simulink model "TemplateLgV2"  (Simulink 7.3)
settings: Solver=ode5  StartTime=0.0  StopTime=inf  FixedStep=0.1  RelTol=1e-3
undefined symbols (not defined in the file): eta1_0_real, v1_0_real, velocitySatValues1
libraries: simulink x23, dspmtrx3 x18, marine_gnc x9, dspindex x5, simulink_extras x1, dspinverses x1
(part 4 of 4)

== system TemplateLgV2/Main Subsystems/Guidance/Line-Of-Sight Path-Following/Line-Of-Sight/LOS heading/psi_los^qs = psi_los^sq ==
  epsilon_n : Inport
  Delta : Inport  Port=2
  epsilon_n^s : Inport  Port=3
  epsilon_n^q : Inport  Port=4
  epsilon_n^qs : Inport  Port=5
  ( )^2 : Math  Operator=square  OutDataType=fixdt(1, 16)  OutScaling=2^0  SaturateOnIntegerOverflow=on
  2 : Gain  Gain=2  ParameterDataType=fixdt(1, 16)  ParameterScaling=2^0  OutDataType=fixdt(1, 16)  OutScaling=2^0
  Add : Sum  Inputs=|++  OutDataType=fixdt(1, 16)  OutScaling=2^-10
  Delta^2 : Math  Operator=square  OutDataType=fixdt(1, 16)  OutScaling=2^0  SaturateOnIntegerOverflow=on
  Divide : Product  Inputs=*/  OutDataType=fixdt(1, 16)  OutScaling=2^-10
  Divide1 : Product  Inputs=*/  OutDataType=fixdt(1, 16)  OutScaling=2^-10
  Product : Product  Inputs=4  Multiplication=Matrix(*)  OutDataType=fixdt(1, 16)  OutScaling=2^0  RndMeth=Zero
  Product1 : Product  Multiplication=Matrix(*)  OutDataType=fixdt(1, 16)  OutScaling=2^0  RndMeth=Zero
  Subtract : Sum  Inputs=|+-  OutDataType=fixdt(1, 16)  OutScaling=2^-10
  epsilon_n^2 : Math  Operator=square  OutDataType=fixdt(1, 16)  OutScaling=2^0  SaturateOnIntegerOverflow=on
  psi_los^qs : Outport
  wires:
  2/1 -> Divide/1
  Divide1/1 -> Subtract/2
  Product1/1 -> Divide1/1
  epsilon_n^qs/1 -> Product1/2
  ( )^2/1 -> Divide/2
  Delta^2/1 -> Add/1
  Add/1 -> Divide1/2, ( )^2/1
  epsilon_n^2/1 -> Add/2
  Product/1 -> 2/1
  epsilon_n^q/1 -> Product/4
  epsilon_n^s/1 -> Product/3
  epsilon_n/1 -> epsilon_n^2/1, Product/2
  Delta/1 -> Product1/1, Delta^2/1, Product/1
  Divide/1 -> Subtract/1
  Subtract/1 -> psi_los^qs/1

== system TemplateLgV2/Main Subsystems/Guidance/Line-Of-Sight Path-Following/Line-Of-Sight/LOS heading/psi_los^s eq ==
  epsilon_n : Inport
  Delta : Inport  Port=2
  psi_d^s : Inport  Port=3
  epsilon_n^s : Inport  Port=4
  Add : Sum  Inputs=|++  OutDataType=fixdt(1, 16)  OutScaling=2^-10
  Delta^2 : Math  Operator=square  OutDataType=fixdt(1, 16)  OutScaling=2^0  SaturateOnIntegerOverflow=on
  Divide : Product  Inputs=*/  OutDataType=fixdt(1, 16)  OutScaling=2^-10
  Product : Product  OutDataType=fixdt(1, 16)  OutScaling=2^0  RndMeth=Zero
  Subtract : Sum  Inputs=|+-  OutDataType=fixdt(1, 16)  OutScaling=2^-10
  epsilon_n^2 : Math  Operator=square  OutDataType=fixdt(1, 16)  OutScaling=2^0  SaturateOnIntegerOverflow=on
  psi_los^s : Outport
  wires:
  Delta/1 -> Divide/1, Delta^2/1
  Delta^2/1 -> Add/1
  Add/1 -> Divide/2
  epsilon_n^2/1 -> Add/2
  epsilon_n/1 -> epsilon_n^2/1
  Subtract/1 -> psi_los^s/1
  Product/1 -> Subtract/2
  psi_d^s/1 -> Subtract/1
  epsilon_n^s/1 -> Product/2
  Divide/1 -> Product/1

== system TemplateLgV2/Main Subsystems/Guidance/Line-Of-Sight Path-Following/Line-Of-Sight/LOS heading/psi_los^s^2 eq ==
  epsilon_n : Inport
  Delta : Inport  Port=2
  epsilon_n^s : Inport  Port=3
  psi_d¨^s^2 : Inport  Port=4
  epsilon_n^s^2 : Inport  Port=5
  ( )^2 : Math  Operator=square  OutDataType=fixdt(1, 16)  OutScaling=2^0  SaturateOnIntegerOverflow=on
  (epsilon_n^s)^2 : Math  Operator=square  OutDataType=fixdt(1, 16)  OutScaling=2^0  SaturateOnIntegerOverflow=on
  2 : Gain  Gain=2  ParameterDataType=fixdt(1, 16)  ParameterScaling=2^0  OutDataType=fixdt(1, 16)  OutScaling=2^0
  Add : Sum  Inputs=|++  OutDataType=fixdt(1, 16)  OutScaling=2^-10
  Delta^2 : Math  Operator=square  OutDataType=fixdt(1, 16)  OutScaling=2^0  SaturateOnIntegerOverflow=on
  Divide : Product  Inputs=*/  OutDataType=fixdt(1, 16)  OutScaling=2^-10
  Divide1 : Product  Inputs=*/  OutDataType=fixdt(1, 16)  OutScaling=2^-10
  Product : Product  Inputs=3  Multiplication=Matrix(*)  OutDataType=fixdt(1, 16)  OutScaling=2^0  RndMeth=Zero
  Product1 : Product  Multiplication=Matrix(*)  OutDataType=fixdt(1, 16)  OutScaling=2^0  RndMeth=Zero
  Sum : Sum  Inputs=++-  OutDataType=fixdt(1, 16)  OutScaling=2^-10
  epsilon_n^2 : Math  Operator=square  OutDataType=fixdt(1, 16)  OutScaling=2^0  SaturateOnIntegerOverflow=on
  psi_los^s^2 : Outport
  wires:
  epsilon_n^s^2/1 -> Product1/2
  epsilon_n^s/1 -> (epsilon_n^s)^2/1
  2/1 -> Divide/1
  Divide1/1 -> Sum/3
  Product1/1 -> Divide1/1
  ( )^2/1 -> Divide/2
  Delta^2/1 -> Add/1
  Add/1 -> Divide1/2, ( )^2/1
  epsilon_n^2/1 -> Add/2
  Product/1 -> 2/1
  (epsilon_n^s)^2/1 -> Product/3
  epsilon_n/1 -> epsilon_n^2/1, Product/2
  Delta/1 -> Product1/1, Delta^2/1, Product/1
  Divide/1 -> Sum/2
  psi_d¨^s^2/1 -> Sum/1
  Sum/1 -> psi_los^s^2/1

== system TemplateLgV2/Main Subsystems/Guidance/Line-Of-Sight Path-Following/Line-Of-Sight/Position error signals/R_2 ==
  psi_d : Inport
  Mux : Mux
  R11 : Trigonometry  Operator=cos
  R12 : Gain  Gain=-1  ParameterDataType=fixdt(1, 16)  ParameterScaling=2^0  OutDataType=fixdt(1, 16)  OutScaling=2^0
  R21 : Trigonometry
  R22 : Gain  ParameterDataType=fixdt(1, 16)  ParameterScaling=2^0  OutDataType=fixdt(1, 16)  OutScaling=2^0
  R_2(psi_d) : Reshape  OutputDimensionality=Customize  OutputDimensions=[2,2]
  R_2 : Outport
  wires:
  R22/1 -> Mux/4
  R12/1 -> Mux/3
  R11/1 -> R22/1, Mux/1
  psi_d/1 -> R11/1, R21/1
  R21/1 -> Mux/2, R12/1
  Mux/1 -> R_2(psi_d)/1
  R_2(psi_d)/1 -> R_2/1

== system TemplateLgV2/Main Subsystems/Guidance/Line-Of-Sight Path-Following/Line-Of-Sight/Position error signals/S_2 ==
  psi_d^s : Inport
  0 : Constant  Value=0  OutDataType=fixdt(1, 16)  OutScaling=2^0
  Mux : Mux
  S12 : Gain  Gain=-1  ParameterDataType=fixdt(1, 16)  ParameterScaling=2^0  OutDataType=fixdt(1, 16)  OutScaling=2^0
  S_2(psi_d^s) : Reshape  OutputDimensionality=Customize  OutputDimensions=[2,2]
  S_2 : Outport
  wires:
  0/1 -> Mux/1, Mux/4
  S12/1 -> Mux/3
  psi_d^s/1 -> Mux/2, S12/1
  Mux/1 -> S_2(psi_d^s)/1
  S_2(psi_d^s)/1 -> S_2/1

== system TemplateLgV2/Main Subsystems/Guidance/Line-Of-Sight Path-Following/Line-Of-Sight/Position error signals/S_2(psi_d^s^2) ==
  psi_d^s^2 : Inport
  0 : Constant  Value=0  OutDataType=fixdt(1, 16)  OutScaling=2^0
  Mux : Mux
  S12 : Gain  Gain=-1  ParameterDataType=fixdt(1, 16)  ParameterScaling=2^0  OutDataType=fixdt(1, 16)  OutScaling=2^0
  S_2(psi_d^s^2) : Reshape  OutputDimensionality=Customize  OutputDimensions=[2,2]
  S_2 : Outport
  wires:
  S_2(psi_d^s^2)/1 -> S_2/1
  Mux/1 -> S_2(psi_d^s^2)/1
  psi_d^s^2/1 -> S12/1, Mux/2
  S12/1 -> Mux/3
  0/1 -> Mux/4, Mux/1

== system TemplateLgV2/Main Subsystems/Guidance/Line-Of-Sight Path-Following/Line-Of-Sight/Position error signals/epsilon^qs = epsilon^sq ==
  R_2^T : Inport
  S_2^T : Inport  Port=2
  Product1 : Product  Multiplication=Matrix(*)  OutDataType=fixdt(1, 16)  OutScaling=2^0  RndMeth=Zero
  epsilon^qs : Outport
  wires:
  R_2^T/1 -> Product1/2
  S_2^T/1 -> Product1/1
  Product1/1 -> epsilon^qs/1

== system TemplateLgV2/Main Subsystems/Guidance/Line-Of-Sight Path-Following/Line-Of-Sight/Position error signals/epsilon^s eq ==
  q - p_d : Inport
  R_2^T : Inport  Port=2
  S_2^T : Inport  Port=3
  p_d^s : Inport  Port=4
  Product : Product  Inputs=3  Multiplication=Matrix(*)  OutDataType=fixdt(1, 16)  OutScaling=2^0  RndMeth=Zero
  Product1 : Product  Multiplication=Matrix(*)  OutDataType=fixdt(1, 16)  OutScaling=2^0  RndMeth=Zero
  Subtract1 : Sum  Inputs=+-  OutDataType=fixdt(1, 16)  OutScaling=2^-10
  epsilon^s : Outport
  wires:
  q - p_d/1 -> Product/3
  Subtract1/1 -> epsilon^s/1
  Product1/1 -> Subtract1/2
  Product/1 -> Subtract1/1
  p_d^s/1 -> Product1/2
  R_2^T/1 -> Product1/1, Product/2
  S_2^T/1 -> Product/1

== system TemplateLgV2/Main Subsystems/Guidance/Line-Of-Sight Path-Following/Line-Of-Sight/Position error signals/epsilon^s^2 eq ==
  q - p_d : Inport
  p_d^s : Inport  Port=2
  R_2^T : Inport  Port=3
  S_2^T : Inport  Port=4
  S_2(psi_d^s^2)^T : Inport  Port=5
  p_d^s^2 : Inport  Port=6
  2 : Gain  Gain=2  ParameterDataType=fixdt(1, 16)  ParameterScaling=2^0  OutDataType=fixdt(1, 16)  OutScaling=2^0
  Add : Sum  OutDataType=fixdt(1, 16)  OutScaling=2^-10
  Gain : Gain  ParameterDataType=fixdt(1, 16)  ParameterScaling=2^0  OutDataType=fixdt(1, 16)  OutScaling=2^0
  Product : Product  Multiplication=Matrix(*)  OutDataType=fixdt(1, 16)  OutScaling=2^0  RndMeth=Zero
  Product1 : Product  Inputs=3  Multiplication=Matrix(*)  OutDataType=fixdt(1, 16)  OutScaling=2^0  RndMeth=Zero
  Product2 : Product  Inputs=3  Multiplication=Matrix(*)  OutDataType=fixdt(1, 16)  OutScaling=2^0  RndMeth=Zero
  Product3 : Product  Multiplication=Matrix(*)  OutDataType=fixdt(1, 16)  OutScaling=2^0  RndMeth=Zero
  Sum : Sum  Inputs=+--  OutDataType=fixdt(1, 16)  OutScaling=2^-10
  epsilon^s^2 : Outport
  wires:
  Product3/1 -> Sum/3
  p_d^s^2/1 -> Product3/2
  p_d^s/1 -> Product2/3
  2/1 -> Sum/2
  Product1/1 -> Sum/1
  q - p_d/1 -> Product1/3
  R_2^T/1 -> Product3/1, Product2/2, Product1/2
  Add/1 -> Product1/1
  Product/1 -> Add/2
  S_2^T/1 -> Product/2, Product2/1, Product/1
  S_2(psi_d^s^2)^T/1 -> Add/1
  Gain/1 -> epsilon^s^2/1
  Product2/1 -> 2/1
  Sum/1 -> Gain/1

== system TemplateLgV2/Main Subsystems/Guidance/Line-Of-Sight Path-Following/Path/Ellipse path/p_d eq ==
  s : Inport
  r_x : Inport  Port=2
  r_y : Inport  Port=3
  origo_x : Inport  Port=4
  origo_y : Inport  Port=5
  k : Inport  Port=6
  Add : Sum  OutDataType=fixdt(1, 16)  OutScaling=2^-10
  Add1 : Sum  OutDataType=fixdt(1, 16)  OutScaling=2^-10
  Mux1 : Mux  Inputs=2
  Product : Product  OutDataType=fixdt(1, 16)  OutScaling=2^0  RndMeth=Zero
  Product1 : Product  OutDataType=fixdt(1, 16)  OutScaling=2^0  RndMeth=Zero
  Product2 : Product  OutDataType=fixdt(1, 16)  OutScaling=2^0  RndMeth=Zero
  cos(s) : Trigonometry  Operator=cos
  sin(s) : Trigonometry
  p_d : Outport
  wires:
  Product2/1 -> sin(s)/1, cos(s)/1
  k/1 -> Product2/2
  s/1 -> Product2/1
  Add1/1 -> Mux1/2
  Product1/1 -> Add1/1
  Product/1 -> Add/1
  origo_y/1 -> Add1/2
  origo_x/1 -> Add/2
  Mux1/1 -> p_d/1
  r_y/1 -> Product1/1
  r_x/1 -> Product/1
  Add/1 -> Mux1/1
  sin(s)/1 -> Product1/2
  cos(s)/1 -> Product/2

== system TemplateLgV2/Main Subsystems/Guidance/Line-Of-Sight Path-Following/Path/Ellipse path/p_d^s eq ==
  s : Inport
  r_x : Inport  Port=2
  r_y : Inport  Port=3
  k : Inport  Port=4
  Gain : Gain  Gain=-1  ParameterDataType=fixdt(1, 16)  ParameterScaling=2^0  OutDataType=fixdt(1, 16)  OutScaling=2^0
  Mux1 : Mux  Inputs=2
  Product : Product  Inputs=3  OutDataType=fixdt(1, 16)  OutScaling=2^0  RndMeth=Zero
  Product1 : Product  Inputs=3  OutDataType=fixdt(1, 16)  OutScaling=2^0  RndMeth=Zero
  Product2 : Product  OutDataType=fixdt(1, 16)  OutScaling=2^0  RndMeth=Zero
  cos(s) : Trigonometry  Operator=cos
  sin(s) : Trigonometry
  p_d^s : Outport
  wires:
  Product2/1 -> sin(s)/1, cos(s)/1
  k/1 -> Product/3, Product1/3, Product2/2
  Mux1/1 -> p_d^s/1
  r_y/1 -> Product1/1
  r_x/1 -> Product/1
  Product1/1 -> Mux1/2
  Gain/1 -> Mux1/1
  Product/1 -> Gain/1
  cos(s)/1 -> Product1/2
  sin(s)/1 -> Product/2
  s/1 -> Product2/1

== system TemplateLgV2/Main Subsystems/Guidance/Line-Of-Sight Path-Following/Path/Ellipse path/p_d^s^2 eq ==
  s : Inport
  r_x : Inport  Port=2
  r_y : Inport  Port=3
  k : Inport  Port=4
  Gain : Gain  Gain=-1  ParameterDataType=fixdt(1, 16)  ParameterScaling=2^0  OutDataType=fixdt(1, 16)  OutScaling=2^0
  Gain1 : Gain  Gain=-1  ParameterDataType=fixdt(1, 16)  ParameterScaling=2^0  OutDataType=fixdt(1, 16)  OutScaling=2^0
  Math Function : Math  Operator=square  OutDataType=fixdt(1, 16)  OutScaling=2^0  SaturateOnIntegerOverflow=on
  Mux2 : Mux  Inputs=2
  Product : Product  Inputs=3  OutDataType=fixdt(1, 16)  OutScaling=2^0  RndMeth=Zero
  Product1 : Product  Inputs=3  OutDataType=fixdt(1, 16)  OutScaling=2^0  RndMeth=Zero
  Product2 : Product  OutDataType=fixdt(1, 16)  OutScaling=2^0  RndMeth=Zero
  cos(s) : Trigonometry  Operator=cos
  sin(s) : Trigonometry
  p_d^s^2 : Outport
  wires:
  Math Function/1 -> Product/3, Product1/3
  Product2/1 -> sin(s)/1, cos(s)/1
  s/1 -> Product2/1
  k/1 -> Math Function/1, Product2/2
  r_x/1 -> Product/1
  r_y/1 -> Product1/1
  Mux2/1 -> p_d^s^2/1
  sin(s)/1 -> Product1/2
  cos(s)/1 -> Product/2
  Gain1/1 -> Mux2/2
  Product1/1 -> Gain1/1
  Gain/1 -> Mux2/1
  Product/1 -> Gain/1

== system TemplateLgV2/Main Subsystems/Guidance/Line-Of-Sight Path-Following/Path/Ellipse path/p_d^s^3 eq ==
  s : Inport
  r_x : Inport  Port=2
  r_y : Inport  Port=3
  k : Inport  Port=4
  Constant : Constant  Value=3  OutDataType=fixdt(1, 16)  OutScaling=2^0
  Gain : Gain  Gain=-1  ParameterDataType=fixdt(1, 16)  ParameterScaling=2^0  OutDataType=fixdt(1, 16)  OutScaling=2^0
  Math Function : Math  Operator=pow  OutDataType=fixdt(1, 16)  OutScaling=2^0  SaturateOnIntegerOverflow=on
  Mux3 : Mux  Inputs=2
  Product : Product  Inputs=3  OutDataType=fixdt(1, 16)  OutScaling=2^0  RndMeth=Zero
  Product1 : Product  Inputs=3  OutDataType=fixdt(1, 16)  OutScaling=2^0  RndMeth=Zero
  Product2 : Product  OutDataType=fixdt(1, 16)  OutScaling=2^0  RndMeth=Zero
  cos(s)3 : Trigonometry  Operator=cos
  sin(s)3 : Trigonometry
  p_d^s^3 : Outport
  wires:
  Math Function/1 -> Product/3, Product1/3
  Constant/1 -> Math Function/2
  Product2/1 -> cos(s)3/1, sin(s)3/1
  s/1 -> Product2/1
  k/1 -> Math Function/1, Product2/2
  r_y/1 -> Product1/1
  r_x/1 -> Product/1
  sin(s)3/1 -> Product/2
  cos(s)3/1 -> Product1/2
  Product/1 -> Mux3/1
  Mux3/1 -> p_d^s^3/1
  Gain/1 -> Mux3/2
  Product1/1 -> Gain/1

== system TemplateLgV2/Main Subsystems/Guidance/Line-Of-Sight Path-Following/Path/Ellipse path/|p_d^s| eq ==
  p_d^s : Inport
  Product : Product  Multiplication=Matrix(*)  OutDataType=fixdt(1, 16)  OutScaling=2^0  RndMeth=Zero
  p_d^s^T : dspmtrx3/Transpose  SystemSampleTime=-1  Hermitian=off  overflowFlag=off
  sqrt : Math  Operator=sqrt  OutDataType=fixdt(1, 16)  OutScaling=2^0  SaturateOnIntegerOverflow=on
  |p_d^s| : Outport
  wires:
  p_d^s^T/1 -> Product/1
  Product/1 -> sqrt/1
  sqrt/1 -> |p_d^s|/1
  p_d^s/1 -> p_d^s^T/1, Product/2

== system TemplateLgV2/Main Subsystems/Guidance/Line-Of-Sight Path-Following/Path/Path Switch workaround + limiter/Limiter ==
  p_d : Inport  OutDataType=sfix(16)  OutScaling=2^0
  Demux : Demux  Outputs=2
  Mux1 : Mux  Inputs=2
  Saturation x : simulink/Discontinuities/Saturation Dynamic  SystemSampleTime=-1  OutMin=[]  OutMax=[]  OutDataTypeStr=Inherit: Same as second input  OutDataType=fixdt(1, 16)  OutScaling=2^-10  DoSatur=off
  Saturation y : simulink/Discontinuities/Saturation Dynamic  SystemSampleTime=-1  OutMin=[]  OutMax=[]  OutDataTypeStr=Inherit: Same as second input  OutDataType=fixdt(1, 16)  OutScaling=2^-10  DoSatur=off
  sat_p_d : Outport  PortDimensions=2  OutDataType=sfix(16)  OutScaling=2^0
  wires:
  Saturation y/1 -> Mux1/2
  Saturation x/1 -> Mux1/1
  Demux/2 -> Saturation y/2
  Demux/1 -> Saturation x/2
  p_d/1 -> Demux/1
  Mux1/1 -> sat_p_d/1
  [xdmax] -> Saturation x/1
  [xdmin] -> Saturation x/3
  [ydmax] -> Saturation y/1
  [ydmin] -> Saturation y/3

== system TemplateLgV2/Main Subsystems/Guidance/Line-Of-Sight Path-Following/Path/Path Switch workaround + limiter/p_d selcetor ==
  note: Path Selector == 1: Linear path
      | Path Selector == 0: Ellipse path
  Path Selector : Inport  OutDataType=fixdt(1, 16)  OutScaling=2^0
  Add : Sum  OutDataType=fixdt(1, 16)  OutScaling=2^-10
  Constant : Constant  OutDataType=fixdt(1, 16)  OutScaling=2^0
  Product : Product  OutDataType=fixdt(1, 16)  OutScaling=2^0  RndMeth=Zero
  Product1 : Product  OutDataType=fixdt(1, 16)  OutScaling=2^0  RndMeth=Zero
  Subract : Sum  Inputs=+-  OutDataType=fixdt(1, 16)  OutScaling=2^-10
  p_d : Outport
  wires:
  Add/1 -> p_d/1
  Path Selector/1 -> Product/2, Subract/2  "chosen path"
  Constant/1 -> Subract/1
  Product/1 -> Add/1
  Subract/1 -> Product1/2
  Product1/1 -> Add/2
  [pdLinear] -> Product/1
  [pdEllipse] -> Product1/1

== system TemplateLgV2/Main Subsystems/Guidance/Line-Of-Sight Path-Following/Path/Path Switch workaround + limiter/p_d^s selcetor ==
  note: Path Selector == 1: Linear path
      | Path Selector == 0: Ellipse path
  Path Selector : Inport  OutDataType=fixdt(1, 16)  OutScaling=2^0
  Add : Sum  OutDataType=fixdt(1, 16)  OutScaling=2^-10
  Constant : Constant  OutDataType=fixdt(1, 16)  OutScaling=2^0
  Product : Product  OutDataType=fixdt(1, 16)  OutScaling=2^0  RndMeth=Zero
  Product1 : Product  OutDataType=fixdt(1, 16)  OutScaling=2^0  RndMeth=Zero
  Subract : Sum  Inputs=+-  OutDataType=fixdt(1, 16)  OutScaling=2^-10
  p_d^s : Outport
  wires:
  [pd_sEllipse] -> Product1/1
  [pd_sLinear] -> Product/1
  Product1/1 -> Add/2
  Subract/1 -> Product1/2
  Product/1 -> Add/1
  Constant/1 -> Subract/1
  Path Selector/1 -> Subract/2, Product/2  "chosen path"
  Add/1 -> p_d^s/1

== system TemplateLgV2/Main Subsystems/Guidance/Line-Of-Sight Path-Following/Path/Path Switch workaround + limiter/p_d^s^2 selcetor ==
  note: Path Selector == 1: Linear path
      | Path Selector == 0: Ellipse path
  Path Selector : Inport  OutDataType=fixdt(1, 16)  OutScaling=2^0
  Add : Sum  OutDataType=fixdt(1, 16)  OutScaling=2^-10
  Constant : Constant  OutDataType=fixdt(1, 16)  OutScaling=2^0
  Product : Product  OutDataType=fixdt(1, 16)  OutScaling=2^0  RndMeth=Zero
  Product1 : Product  OutDataType=fixdt(1, 16)  OutScaling=2^0  RndMeth=Zero
  Subract : Sum  Inputs=+-  OutDataType=fixdt(1, 16)  OutScaling=2^-10
  p_d^s^2 : Outport
  wires:
  Add/1 -> p_d^s^2/1
  Path Selector/1 -> Product/2, Subract/2  "chosen path"
  Constant/1 -> Subract/1
  Product/1 -> Add/1
  Subract/1 -> Product1/2
  Product1/1 -> Add/2
  [pd_s_2Linear] -> Product/1
  [pd_s_2Ellipse] -> Product1/1

== system TemplateLgV2/Main Subsystems/Guidance/Line-Of-Sight Path-Following/Path/Path Switch workaround + limiter/p_d^s^3 selcetor ==
  note: Path Selector == 1: Linear path
      | Path Selector == 0: Ellipse path
  Path Selector : Inport  OutDataType=fixdt(1, 16)  OutScaling=2^0
  Add : Sum  OutDataType=fixdt(1, 16)  OutScaling=2^-10
  Constant : Constant  OutDataType=fixdt(1, 16)  OutScaling=2^0
  Product : Product  OutDataType=fixdt(1, 16)  OutScaling=2^0  RndMeth=Zero
  Product1 : Product  OutDataType=fixdt(1, 16)  OutScaling=2^0  RndMeth=Zero
  Subract : Sum  Inputs=+-  OutDataType=fixdt(1, 16)  OutScaling=2^-10
  p_d^s^3 : Outport
  wires:
  [pd_s_3Ellipse] -> Product1/1
  [pd_s_3Linear] -> Product/1
  Product1/1 -> Add/2
  Subract/1 -> Product1/2
  Product/1 -> Add/1
  Constant/1 -> Subract/1
  Path Selector/1 -> Subract/2, Product/2  "chosen path"
  Add/1 -> p_d^s^3/1

== system TemplateLgV2/Main Subsystems/Guidance/Line-Of-Sight Path-Following/Path/Path Switch workaround + limiter/p_d^s^3 selcetor1 ==
  note: Path Selector == 1: Linear path
      | Path Selector == 0: Ellipse path
  Path Selector : Inport  OutDataType=fixdt(1, 16)  OutScaling=2^0
  Add : Sum  OutDataType=fixdt(1, 16)  OutScaling=2^-10
  Constant : Constant  OutDataType=fixdt(1, 16)  OutScaling=2^0
  Product : Product  OutDataType=fixdt(1, 16)  OutScaling=2^0  RndMeth=Zero
  Product1 : Product  OutDataType=fixdt(1, 16)  OutScaling=2^0  RndMeth=Zero
  Subract : Sum  Inputs=+-  OutDataType=fixdt(1, 16)  OutScaling=2^-10
  |p_d^s| : Outport
  wires:
  Add/1 -> |p_d^s|/1
  Path Selector/1 -> Product/2, Subract/2  "chosen path"
  Constant/1 -> Subract/1
  Product/1 -> Add/1
  Subract/1 -> Product1/2
  Product1/1 -> Add/2
  [pd_sabsLinear] -> Product/1
  [pd_sabsEllipse] -> Product1/1

== system TemplateLgV2/Main Subsystems/Guidance/Line-Of-Sight Path-Following/Path/Straight path/p_d eq ==
  s : Inport
  x_1 : Inport  Port=2
  y_1 : Inport  Port=3
  x_2 : Inport  Port=4
  y_2 : Inport  Port=5
  (x_2 - x_1) * s : Product  OutDataType=fixdt(1, 16)  OutScaling=2^0  RndMeth=Zero
  (x_2 - x_1) * s + x_1 : Sum  OutDataType=fixdt(1, 16)  OutScaling=2^-10
  (y_2 - y_1) * s : Product  OutDataType=fixdt(1, 16)  OutScaling=2^0  RndMeth=Zero
  (y_2 - y_1) * s + y_1 : Sum  OutDataType=fixdt(1, 16)  OutScaling=2^-10
  Mux1 : Mux  Inputs=2
  x_2 - x_1 : Sum  Inputs=+-  OutDataType=fixdt(1, 16)  OutScaling=2^-10
  y_2 - y_1 : Sum  Inputs=+-  OutDataType=fixdt(1, 16)  OutScaling=2^-10
  p_d : Outport
  wires:
  Mux1/1 -> p_d/1
  y_1/1 -> (y_2 - y_1) * s + y_1/2, y_2 - y_1/2
  y_2/1 -> y_2 - y_1/1
  x_1/1 -> (x_2 - x_1) * s + x_1/2, x_2 - x_1/2
  x_2/1 -> x_2 - x_1/1
  s/1 -> (y_2 - y_1) * s/2, (x_2 - x_1) * s/2
  y_2 - y_1/1 -> (y_2 - y_1) * s/1
  x_2 - x_1/1 -> (x_2 - x_1) * s/1
  (y_2 - y_1) * s/1 -> (y_2 - y_1) * s + y_1/1
  (x_2 - x_1) * s/1 -> (x_2 - x_1) * s + x_1/1
  (y_2 - y_1) * s + y_1/1 -> Mux1/2
  (x_2 - x_1) * s + x_1/1 -> Mux1/1

== system TemplateLgV2/Main Subsystems/Guidance/Line-Of-Sight Path-Following/Path/Straight path/p_d^s eq ==
  x_1 : Inport
  y_1 : Inport  Port=2
  x_2 : Inport  Port=3
  y_2 : Inport  Port=4
  Mux1 : Mux  Inputs=2
  x_2 - x_1 : Sum  Inputs=+-  OutDataType=fixdt(1, 16)  OutScaling=2^-10
  y_2 - y_1 : Sum  Inputs=+-  OutDataType=fixdt(1, 16)  OutScaling=2^-10
  p_d^s : Outport
  wires:
  y_1/1 -> y_2 - y_1/2
  y_2/1 -> y_2 - y_1/1
  x_1/1 -> x_2 - x_1/2
  x_2/1 -> x_2 - x_1/1
  y_2 - y_1/1 -> Mux1/2
  x_2 - x_1/1 -> Mux1/1
  Mux1/1 -> p_d^s/1

== system TemplateLgV2/Main Subsystems/Guidance/Line-Of-Sight Path-Following/Path/Straight path/|p_d^s| eq ==
  p_d^s : Inport
  Product : Product  Multiplication=Matrix(*)  OutDataType=fixdt(1, 16)  OutScaling=2^0  RndMeth=Zero
  p_d^s^T : dspmtrx3/Transpose  SystemSampleTime=-1  Hermitian=off  overflowFlag=off
  sqrt : Math  Operator=sqrt  OutDataType=fixdt(1, 16)  OutScaling=2^0  SaturateOnIntegerOverflow=on
  |p_d^s| : Outport
  wires:
  p_d^s/1 -> Product/2, p_d^s^T/1
  sqrt/1 -> |p_d^s|/1
  Product/1 -> sqrt/1
  p_d^s^T/1 -> Product/1

== system TemplateLgV2/Main Subsystems/Naviagation/Input from SIT/u_act to tau/u_act to f_act/u_1 to f_1 VSP speed 0.3 ==
  note: Table valid for VSP speed == 0.30
  u_1 : Inport
  u_1 to f_1 : Lookup  InputValues=[-1.0000 -0.9500 -0.9000 -0.8500 -0.8000 -0.7500 -0.7000 -0.6500 -0.6000 -0.5500 -0.5000 -0.4500 -0.4000 -0.3500 -0.3000 -0.2500 -0.2000 -0.1500 -0.1000 -0.0500 0 0.0500 0.1000 0.1500 0.2000 0.2500 0.3000 0.3500 0.4000 0.4500 0.5000 0.5500 0.6000 0.6500 0.7000 0.7500 0.8000 0.8500 0.9000]  Table=[-0.6829 -0.6369 -0.5785 -0.5165 -0.4456 -0.3725 -0.3308 -0.2827 -0.2277 -0.1517 -0.1240 -0.0769 -0.0238 0.0039 0.0377 0.0635 0.1051 0.1196 0.1412 0.1721 0.1754 0.1774 0.2104 0.2200 0.2266 0.2673 0.3025 0.3486 0.3896 0.4252 0.4782 0.5164 0.5695 0.6195 0.6723 0.7449 0.7836 0.8414 0.8987 ]  LookUpMeth=Interpolation-Use End Values  OutDataType=fixdt(1, 16)  OutScaling=2^0
  f_1 : Outport
  wires:
  u_1/1 -> u_1 to f_1/1
  u_1 to f_1/1 -> f_1/1

== system TemplateLgV2/Main Subsystems/Naviagation/Input from SIT/u_act to tau/u_act to f_act/u_2 to f_2 VSP speed 0.3 ==
  note: Switching to the lookup table giving the closes value
  note: workaround setup
  note: Tables valid for VSP speed == 0.30
  u_2 : Inport
  Gain1 : Gain  Gain=3  ParameterDataType=fixdt(1, 16)  ParameterScaling=2^0  OutDataType=fixdt(1, 16)  OutScaling=2^0
  If < 0.00391 : simulink/Logic and Bit Operations/Compare To Constant  SystemSampleTime=-1  relop=<  const=-0.5  LogicOutDataTypeMode=uint8
  If < 0.06731 : simulink/Logic and Bit Operations/Compare To Constant  SystemSampleTime=-1  relop=<  const=-0.1  LogicOutDataTypeMode=uint8
  If >= 0.00391 : simulink/Logic and Bit Operations/Compare To Constant  SystemSampleTime=-1  relop=>=  const=-0.5  LogicOutDataTypeMode=uint8
  If >= 0.06731 : simulink/Logic and Bit Operations/Compare To Constant  SystemSampleTime=-1  relop=>=  const=-0.1  LogicOutDataTypeMode=uint8
  Logical Operator : Logic  AllPortsSameDT=off  OutDataTypeMode=boolean  LogicDataType=fixdt(0, 8)  OutDataTypeStr=boolean
  Multiport Switch : MultiPortSwitch  OutDataType=fixdt(1, 16)  OutScaling=2^0
  Sum : Sum  Inputs=+++  OutDataType=fixdt(1, 16)  OutScaling=2^0
  Sum1 : Sum  Inputs=|++  OutDataType=fixdt(1, 16)  OutScaling=2^0
  u_2 < -0.1 && u_2 >= -0.2 : Lookup  InputValues=|  Table=|  LookUpMeth=Interpolation-Use End Values  OutDataType=fixdt(1, 16)  OutScaling=2^0
      InputValues=|
      | [-0.2000
      |    -0.1500
      |    -0.1000]
      Table=|
      | [-0.0105
      |     0.0226
      |     0.0673]
  u_2 < -0.5 : Lookup  InputValues=|  Table=|  LookUpMeth=Interpolation-Use End Values  OutDataType=fixdt(1, 16)  OutScaling=2^0
      InputValues=|
      | [-1.0000
      |    -0.9500
      |    -0.9000
      |    -0.8500
      |    -0.8000
      |    -0.7500
      |    -0.7000
      |    -0.6500
      |    -0.6000
      |    -0.5500
      |    -0.5000]
      Table=|
      | [-0.2704
      |    -0.2259
      |    -0.1903
      |    -0.1697
      |    -0.1518
      |    -0.1234
      |    -0.0994
      |    -0.0817
      |    -0.0612
      |    -0.0123
      |     0.0039]
  u_2 => 0 : Lookup  InputValues=|  Table=|  LookUpMeth=Interpolation-Use End Values  OutDataType=fixdt(1, 16)  OutScaling=2^0
      InputValues=|
      | [0
      |     0.0500
      |     0.1000
      |     0.1500
      |     0.2000
      |     0.2500
      |     0.3000
      |     0.3500
      |     0.4000
      |     0.4500
      |     0.5000
      |     0.5500
      |     0.6000
      |     0.6500
      |     0.7000
      |     0.7500
      |     0.8000
      |     0.8500]
      Table=|
      | [0.0872
      |     0.0930
      |     0.1182
      |     0.1412
      |     0.1892
      |     0.2146
      |     0.2678
      |     0.3096
      |     0.3551
      |     0.4013
      |     0.4566
      |     0.5051
      |     0.5477
      |     0.6060
      |     0.6703
      |     0.7437
      |     0.7604
      |     0.7634]
  f_2 : Outport
  wires:
  Multiport Switch/1 -> f_2/1
  Sum/1 -> Multiport Switch/1
  If >= 0.06731/1 -> Gain1/1
  If < 0.00391/1 -> Sum/1
  u_2/1 -> u_2 < -0.5/1, If >= 0.06731/1, If < 0.00391/1, If >= 0.00391/1, If < 0.06731/1, u_2 => 0/1, u_2 < -0.1 && u_2 >= -0.2/1
  u_2 < -0.5/1 -> Multiport Switch/2
  u_2 => 0/1 -> Multiport Switch/4
  u_2 < -0.1 && u_2 >= -0.2/1 -> Multiport Switch/3
  If < 0.06731/1 -> Logical Operator/2
  If >= 0.00391/1 -> Logical Operator/1
  Gain1/1 -> Sum/3
  Sum1/1 -> Sum/2
  Logical Operator/1 -> Sum1/1, Sum1/2

== system TemplateLgV2/Main Subsystems/Naviagation/Input from SIT/u_act to tau/u_act to f_act/u_3 to f_3 VSP speed 0.3 ==
  note: Table valid for VSP speed == 0.30
  u_3 : Inport
  u_3 to f_3 : Lookup  InputValues=[-1.0000,-0.9500,-0.9000,-0.8500,-0.8000,-0.7500,-0.7000,-0.6500,-0.6000,-0.5500,-0.5000,-0.4500,-0.4000,-0.3500,-0.3000,-0.2000,-0.1500,-0.1000,-0.0500,0,0.0500,0.1000,0.1500,0.2000,0.2500,0.3000,0.3500,0.4000,0.4500,0.5000,0.5500,0.6000,0.6500,0.7000,0.7500,0.8000,0.8500,0.9500,1.0000]  Table=[-0.5408,-0.5036,-0.4487,-0.3802,-0.3147,-0.2525,-0.2338,-0.1568,-0.1034,-0.0647,-0.0054,0.0221,0.0572,0.0747,0.0991,0.1258,0.1385,0.1447,0.1539,0.1625,0.1712,0.1976,0.2258,0.2443,0.3058,0.3460,0.3989,0.4342,0.4932,0.5524,0.5814,0.6394,0.6851,0.7496,0.8081,0.8382,0.8665,0.8767,0.8885]  LookUpMeth=Interpolation-Use End Values  OutDataType=fixdt(1, 16)  OutScaling=2^0
  f_3 : Outport
  wires:
  u_3/1 -> u_3 to f_3/1
  u_3 to f_3/1 -> f_3/1

== system TemplateLgV2/Main Subsystems/Naviagation/Input from SIT/u_act to tau/u_act to f_act/u_4 to f_4 VSP speed 0.3 ==
  note: Tables valid for VSP speed == 0.30
  u_4 : Inport
  Gain : Gain  Gain=2  ParameterDataType=fixdt(1, 16)  ParameterScaling=2^0  OutDataType=fixdt(1, 16)  OutScaling=2^0
  If < 0.0451 : simulink/Logic and Bit Operations/Compare To Constant  SystemSampleTime=-1  relop=<  const=-0.1  LogicOutDataTypeMode=uint8
  If >= 0.0451 : simulink/Logic and Bit Operations/Compare To Constant  SystemSampleTime=-1  relop=>=  const=-0.1  LogicOutDataTypeMode=uint8
  Multiport Switch : MultiPortSwitch  Inputs=2  OutDataType=fixdt(1, 16)  OutScaling=2^0
  Sum : Sum  Inputs=+|+  OutDataType=fixdt(1, 16)  OutScaling=2^0
  u_4 < -0.1 : Lookup  InputValues=|  Table=|  LookUpMeth=Interpolation-Use End Values  OutDataType=fixdt(1, 16)  OutScaling=2^0
      InputValues=|
      | [-0.8000
      |    -0.7500
      |    -0.7000
      |    -0.6500
      |    -0.6000
      |    -0.5500
      |    -0.5000
      |    -0.4500
      |    -0.4000
      |    -0.3500
      |    -0.3000
      |    -0.2500
      |    -0.2000
      |    -0.1500
      |    -0.1000]
      Table=|
      | [-0.5212
      |    -0.5163
      |    -0.4943
      |    -0.4390
      |    -0.3803
      |    -0.3603
      |    -0.3132
      |    -0.2567
      |    -0.2102
      |    -0.1609
      |    -0.1267
      |    -0.0819
      |    -0.0554
      |     0.0099
      |     0.0450]
  u_4 >= -0.1 : Lookup  InputValues=|  Table=|  LookUpMeth=Interpolation-Use End Values  OutDataType=fixdt(1, 16)  OutScaling=2^0
      InputValues=|
      | [0.0431
      |     0.0808
      |     0.0867
      |     0.1337
      |     0.1726
      |     0.1963
      |     0.2088
      |     0.2323
      |     0.2969
      |     0.3134
      |     0.3376
      |     0.3743
      |     0.4276]
      Table=|
      | [0.4000
      |     0.4500
      |     0.5000
      |     0.5500
      |     0.6000
      |     0.6500
      |     0.7000
      |     0.7500
      |     0.8000
      |     0.8500
      |     0.9000
      |     0.9500
      |     1.0000]
  f_4 : Outport
  wires:
  Multiport Switch/1 -> f_4/1
  Gain/1 -> Sum/2
  Sum/1 -> Multiport Switch/1
  If >= 0.0451/1 -> Gain/1
  If < 0.0451/1 -> Sum/1
  u_4/1 -> u_4 < -0.1/1, u_4 >= -0.1/1, If >= 0.0451/1, If < 0.0451/1
  u_4 < -0.1/1 -> Multiport Switch/2
  u_4 >= -0.1/1 -> Multiport Switch/3

== system TemplateLgV2/Main Subsystems/Naviagation/Input from SIT/u_act to tau/u_act to f_act/u_5 to f_5 BT power 0.4 ==
  note: If < 0: control input is 1
      | if = 0 control input is 2
      | if > 0: control input is 3
  note: Check if the input value is less, equal or greater then zero
  note: The mapping is divided into 3 parts:
      | Negative, zero and positive
  u_5 : Inport
  Dead Zone +-0.01 : DeadZone  LowerValue=-0.01  UpperValue=0.01  SaturateOnIntegerOverflow=on
  Gain : Gain  Gain=2  ParameterDataType=fixdt(1, 16)  ParameterScaling=2^0  OutDataType=fixdt(1, 16)  OutScaling=2^0
  Gain1 : Gain  Gain=3  ParameterDataType=fixdt(1, 16)  ParameterScaling=2^0  OutDataType=fixdt(1, 16)  OutScaling=2^0
  If < 0 : simulink/Logic and Bit Operations/Compare To Constant  SystemSampleTime=-1  relop=<  const=0  LogicOutDataTypeMode=uint8
  If > 0 : simulink/Logic and Bit Operations/Compare To Constant  SystemSampleTime=-1  relop=>  const=0  LogicOutDataTypeMode=uint8
  Multiport Switch : MultiPortSwitch  OutDataType=fixdt(1, 16)  OutScaling=2^0
  Sum : Sum  Inputs=+++  OutDataType=fixdt(1, 16)  OutScaling=2^0
  if == 0 : simulink/Logic and Bit Operations/Compare To Zero  SystemSampleTime=-1  relop===  LogicOutDataTypeMode=uint8
  u_5 < 0 : Lookup  InputValues=|  Table=|  LookUpMeth=Interpolation-Use End Values  OutDataType=fixdt(1, 16)  OutScaling=2^0
      InputValues=|
      | [-0.2000
      |    -0.1900
      |    -0.1700
      |    -0.1500
      |    -0.1300
      |    -0.1100
      |    -0.0900
      |    -0.0700
      |    -0.0500
      |    -0.0300]
      Table=|
      | [-1.1653
      |    -1.1010
      |    -0.9810
      |    -0.8576
      |    -0.7363
      |    -0.5877
      |    -0.4265
      |    -0.2640
      |    -0.1099
      |     0.0031]
  u_5 = 0 : Constant  Value=0  OutDataType=fixdt(1, 16)  OutScaling=2^0
  u_5 > 0 : Lookup  InputValues=|  Table=|  LookUpMeth=Interpolation-Use End Values  OutDataType=fixdt(1, 16)  OutScaling=2^0
      InputValues=|
      | [0.0300
      |     0.0500
      |     0.0700
      |     0.0900
      |     0.1100
      |     0.1300
      |     0.1500
      |     0.1700
      |     0.1900
      |     0.2000]
      Table=|
      | [0.0103
      |     0.0743
      |     0.1937
      |     0.3232
      |     0.4342
      |     0.5862
      |     0.7291
      |     0.8697
      |     0.9681
      |     1.0229]
  f_5 : Outport
  wires:
  Dead Zone +-0.01/1 -> If > 0/1, if == 0/1, If < 0/1
  u_5 > 0/1 -> Multiport Switch/4
  u_5 = 0/1 -> Multiport Switch/3
  u_5 < 0/1 -> Multiport Switch/2
  u_5/1 -> Dead Zone +-0.01/1, u_5 > 0/1, u_5 < 0/1
  If < 0/1 -> Sum/1
  if == 0/1 -> Gain/1
  If > 0/1 -> Gain1/1
  Sum/1 -> Multiport Switch/1
  Gain/1 -> Sum/2
  Gain1/1 -> Sum/3
  Multiport Switch/1 -> f_5/1

== system TemplateLgV2/Main Subsystems/Guidance/Line-Of-Sight Path-Following/Line-Of-Sight/LOS heading/psi_los eq/rad to [-pi pi] ==
  rad : Inport  OutDataType=sfix(16)  OutScaling=2^0
  Constant : Constant  Value=2*pi  OutDataType=sfix(16)  OutScaling=2^0
  Gain : Gain  Gain=pi  ParameterDataType=sfix(16)  ParameterScaling=2^0  OutDataType=sfix(16)  OutScaling=2^0  SaturateOnIntegerOverflow=on  OutDataTypeStr=Inherit: Same as input  ParamDataTypeStr=Inherit: Same as input
  Math Function : Math  Operator=rem  OutDataType=sfix(16)  OutScaling=2^0  SaturateOnIntegerOverflow=on
  Saturation : Saturate  UpperLimit=1e10  LowerLimit=-1e10
  Sign : Signum
  Sum : Sum  Inputs=|+-  OutDataType=sfix(16)  OutScaling=2^0  SaturateOnIntegerOverflow=on
  Sum1 : Sum  Inputs=|++  OutDataType=sfix(16)  OutScaling=2^0  SaturateOnIntegerOverflow=on
  "[-pi pi]" : Outport  OutDataType=sfix(16)  OutScaling=2^0
  wires:
  Sum/1 -> "[-pi pi]"/1
  Math Function/1 -> Sum/1
  Constant/1 -> Math Function/2
  Sum1/1 -> Math Function/1
  Gain/1 -> Sum1/2, Sum/2
  Sign/1 -> Gain/1
  rad/1 -> Saturation/1
  Saturation/1 -> Sign/1, Sum1/1

== system TemplateLgV2/Main Subsystems/Guidance/Line-Of-Sight Path-Following/Line-Of-Sight/LOS heading/psi_los eq/rad to [-pi pi]1 ==
  rad : Inport  OutDataType=sfix(16)  OutScaling=2^0
  Constant : Constant  Value=2*pi  OutDataType=sfix(16)  OutScaling=2^0
  Gain : Gain  Gain=pi  ParameterDataType=sfix(16)  ParameterScaling=2^0  OutDataType=sfix(16)  OutScaling=2^0  SaturateOnIntegerOverflow=on  OutDataTypeStr=Inherit: Same as input  ParamDataTypeStr=Inherit: Same as input
  Math Function : Math  Operator=rem  OutDataType=sfix(16)  OutScaling=2^0  SaturateOnIntegerOverflow=on
  Saturation : Saturate  UpperLimit=1e10  LowerLimit=-1e10
  Sign : Signum
  Sum : Sum  Inputs=|+-  OutDataType=sfix(16)  OutScaling=2^0  SaturateOnIntegerOverflow=on
  Sum1 : Sum  Inputs=|++  OutDataType=sfix(16)  OutScaling=2^0  SaturateOnIntegerOverflow=on
  "[-pi pi]" : Outport  OutDataType=sfix(16)  OutScaling=2^0
  wires:
  Saturation/1 -> Sum1/1, Sign/1
  rad/1 -> Saturation/1
  Sign/1 -> Gain/1
  Gain/1 -> Sum/2, Sum1/2
  Sum1/1 -> Math Function/1
  Constant/1 -> Math Function/2
  Math Function/1 -> Sum/1
  Sum/1 -> "[-pi pi]"/1

== system TemplateLgV2/Main Subsystems/Guidance/Line-Of-Sight Path-Following/Line-Of-Sight/LOS heading/psi_los eq/rad to [-pi pi]2 ==
  rad : Inport  OutDataType=sfix(16)  OutScaling=2^0
  Constant : Constant  Value=2*pi  OutDataType=sfix(16)  OutScaling=2^0
  Gain : Gain  Gain=pi  ParameterDataType=sfix(16)  ParameterScaling=2^0  OutDataType=sfix(16)  OutScaling=2^0  SaturateOnIntegerOverflow=on  OutDataTypeStr=Inherit: Same as input  ParamDataTypeStr=Inherit: Same as input
  Math Function : Math  Operator=rem  OutDataType=sfix(16)  OutScaling=2^0  SaturateOnIntegerOverflow=on
  Saturation : Saturate  UpperLimit=1e10  LowerLimit=-1e10
  Sign : Signum
  Sum : Sum  Inputs=|+-  OutDataType=sfix(16)  OutScaling=2^0  SaturateOnIntegerOverflow=on
  Sum1 : Sum  Inputs=|++  OutDataType=sfix(16)  OutScaling=2^0  SaturateOnIntegerOverflow=on
  "[-pi pi]" : Outport  OutDataType=sfix(16)  OutScaling=2^0
  wires:
  Sum/1 -> "[-pi pi]"/1
  Math Function/1 -> Sum/1
  Constant/1 -> Math Function/2
  Sum1/1 -> Math Function/1
  Gain/1 -> Sum1/2, Sum/2
  Sign/1 -> Gain/1
  rad/1 -> Saturation/1
  Saturation/1 -> Sign/1, Sum1/1
